simulink model "Satellite_Closed_Loop_Modal_Control"  (R2018b)
settings: Solver=VariableStepAuto  StartTime=0.0  StopTime=200  RelTol=1e-3
values from neighbouring files (symbols this model uses):
  a = 0.5736    [Lab1.m]    (also in Micro_Sat_Open_Loop.m)
  J_r = 0.0004    [Lab1.m]    (also in Micro_Sat_Open_Loop.m)
  J_s = 31.38    [Lab1.m]    (also in Micro_Sat_Open_Loop.m)
  T_e = 0.5    [Lab1.m]    (also in Micro_Sat_Open_Loop.m)
  w = 2.6268    [Lab1.m]    (also in Micro_Sat_Open_Loop.m)
settings Model: Creator=Yavuz  LastModifiedBy=EKOCULU

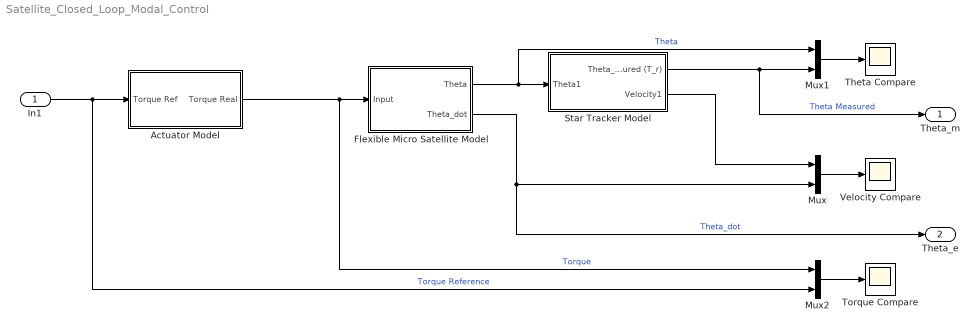
== system Satellite_Closed_Loop_Modal_Control ==
  In1 : Inport
  Actuator Model : Subsystem
  "Flexible Micro Satellite Model " : Subsystem
  Mux : Mux  Inputs=2
  Mux1 : Mux  Inputs=2
  Mux2 : Mux  Inputs=2
  Star Tracker Model : Subsystem
  Theta Compare : Scope
  Torque Compare : Scope
  Velocity Compare : Scope
  Theta_m : Outport
  Theta_e : Outport  Port=2
  wires:
  "Flexible Micro Satellite Model "/1(Theta) -> Star Tracker Model/1(Theta1), Mux1/1  "Theta"
  Actuator Model/1(Torque Real) -> Mux2/1, "Flexible Micro Satellite Model "/1(Input)  "Torque"
  "Flexible Micro Satellite Model "/2(Theta_dot) -> Theta_e/1, Mux/2  "Theta_dot"
  Mux/1 -> Velocity Compare/1
  Mux1/1 -> Theta Compare/1
  Star Tracker Model/1(Theta_measured (T_r)) -> Theta_m/1, Mux1/2  "Theta Measured"
  Mux2/1 -> Torque Compare/1
  In1/1 -> Mux2/2, Actuator Model/1(Torque Ref)  "Torque Reference"
  Star Tracker Model/2(Velocity1) -> Mux/1

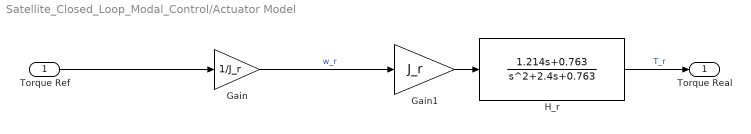
== system Satellite_Closed_Loop_Modal_Control/Actuator Model ==
  Torque Ref : Inport
  Gain : Gain  Gain=1/J_r
  Gain1 : Gain  Gain=J_r
  H_r : TransferFcn  Numerator=[1.214 0.763]  Denominator=[1 2.4 0.763]
  Torque Real : Outport
  wires:
  Torque Ref/1 -> Gain/1
  Gain1/1 -> H_r/1
  H_r/1 -> Torque Real/1  "T_r"
  Gain/1 -> Gain1/1  "w_r"

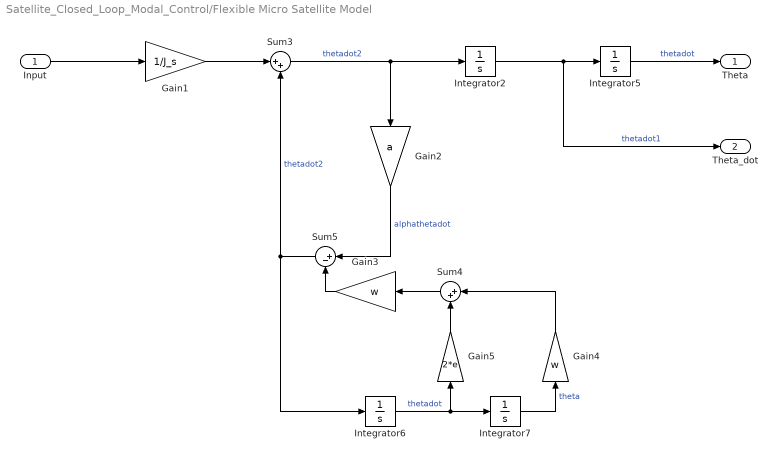
== system Satellite_Closed_Loop_Modal_Control/Flexible Micro Satellite Model  ==
  Input : Inport
  Gain1 : Gain  Gain=1/J_s
  Gain2 : Gain  Gain=a
  Gain3 : Gain  Gain=w
  Gain4 : Gain  Gain=w
  Gain5 : Gain  Gain=2*e
  Integrator{2,5..7} (4 alike) : Integrator
  Sum3 : Sum  Inputs=|++
  Sum4 : Sum  Inputs=|++
  Sum5 : Sum  Inputs=|+-
  Theta : Outport
  Theta_dot : Outport  Port=2
  wires:
  Integrator5/1 -> Theta/1  "thetadot"
  Input/1 -> Gain1/1
  Gain5/1 -> Sum4/2
  Gain3/1 -> Sum5/2
  Integrator2/1 -> Theta_dot/1, Integrator5/1  "thetadot1"
  Gain2/1 -> Sum5/1  "alphathetadot"
  Integrator7/1 -> Gain4/1  "theta"
  Gain1/1 -> Sum3/1
  Sum5/1 -> Integrator6/1, Sum3/2  "thetadot2"
  Integrator6/1 -> Gain5/1, Integrator7/1  "thetadot"
  Sum3/1 -> Gain2/1, Integrator2/1  "thetadot2"
  Sum4/1 -> Gain3/1
  Gain4/1 -> Sum4/1

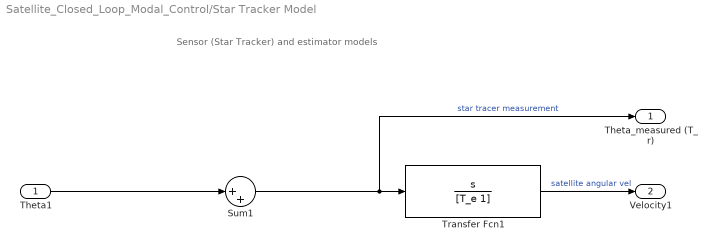
== system Satellite_Closed_Loop_Modal_Control/Star Tracker Model ==
  note: Sensor (Star Tracker) and estimator models
  Theta1 : Inport
  Sum1 : Sum  Inputs=|++
  Transfer Fcn1 : TransferFcn  Numerator=[1 0]  Denominator=[T_e 1]
  Theta_measured (T_r) : Outport
  Velocity1 : Outport  Port=2
  wires:
  Sum1/1 -> Theta_measured (T_r)/1, Transfer Fcn1/1  "star tracer measurement"
  Theta1/1 -> Sum1/1
  Transfer Fcn1/1 -> Velocity1/1  "satellite angular vel"
